simulink model "CryoDetXray"  (R2016b)
settings: Solver=ode45  StartTime=0.0  StopTime=10e-5  MaxStep=Tclk/4  RelTol=1e-3
values from neighbouring files (symbols this model uses):
  Fclk = Fadc    (= 307200000)    [setupCryoFPGAxray.m]
  Tclk = 1/Fclk    (= 3.25520833333e-09)    [setupCryoFPGAxray.m]
undefined symbols (not defined in the file or in its folder): AXI4, Lite, lpf, Naxi, xlipgetpartsetting
libraries: xbsIndex_r4 x1091, CryoDetLib x68, simulink x4, hdlsllib x1
(part 8 of 8)

== system CryoDetXray/DspCore/AdcDac 0/loopFilter1/initial Frequencies ==
  note: initial Frequencies
  note: select initial frequency
      | for now just mux from input registers
      | eventually configure RAM and loading protocol
  channel : Inport
  Gateway Out12 : xbsIndex_r4/Gateway Out  inherit_from_input=off  hdl_port=off  rows=1  columns=1  UseAsDAC=off  DACChannel='1'  interface=None  automatic_assignment=on  address_offset=hex2dec('00')  intf_name=''  intf_description=''  timing_constraint=None  locs_specified=off  LOCs={}  io_standard={}  block_type=gatewayout
  Gateway Out13 : xbsIndex_r4/Gateway Out  inherit_from_input=off  hdl_port=off  rows=1  columns=1  UseAsDAC=off  DACChannel='1'  interface=None  automatic_assignment=on  address_offset=hex2dec('00')  intf_name=''  intf_description=''  timing_constraint=None  locs_specified=off  LOCs={}  io_standard={}  block_type=gatewayout
  Mux : xbsIndex_r4/Mux  inputs=16  en=off  latency=0  precision=Full  arith_type=Unsigned  n_bits=24  bin_pt=24  quantization=Truncate  overflow=Wrap  dbl_ovrd=off  block_type=mux
  initial Freqs : Scope  NumInputPorts=2
  Fi : Outport
  wires:
  channel/1 -> Mux/1, Gateway Out12/1
  [F0] -> Mux/2
  [F1] -> Mux/3
  [F2] -> Mux/4
  [F3] -> Mux/5
  [F4] -> Mux/6
  [F5] -> Mux/7
  [F6] -> Mux/8
  [F7] -> Mux/9
  [F8] -> Mux/10
  [F9] -> Mux/11
  [F10] -> Mux/12
  [F11] -> Mux/13
  Mux/1 -> Gateway Out13/1, Fi/1
  Gateway Out13/1 -> initial Freqs/2
  Gateway Out12/1 -> initial Freqs/1
  [F12] -> Mux/14
  [F13] -> Mux/15
  [F14] -> Mux/16
  [F15] -> Mux/17

== system CryoDetXray/DspCore/AdcDac 0/16LineUDC 0/DAC Sum/DAC Q0 SUM ==
  note: Changed from 12 channel to 16 channels 8Sept2017
  In1 : Inport
  Bus Selector1 : BusSelector  OutputSignals=toDAC0.Q0,toDAC1.Q0,toDAC2.Q0,toDAC3.Q0,toDAC4.Q0,toDAC5.Q0,toDAC6.Q0,toDAC7.Q0,toDAC8.Q0,toDAC9.Q0,toDAC10.Q0,toDAC11.Q0,toDAC12.Q0,toDAC13.Q0,toDAC14.Q0,toDAC15.Q0
  DAC subSum : CryoDetLib/DAC subSum
  Out1 : Outport
  wires:
  In1/1 -> Bus Selector1/1
  Bus Selector1/1 -> DAC subSum/1  "<Q0>"
  Bus Selector1/16 -> DAC subSum/16  "<Q0>"
  DAC subSum/1 -> Out1/1
  Bus Selector1/2 -> DAC subSum/2  "<Q0>"
  Bus Selector1/3 -> DAC subSum/3  "<Q0>"
  Bus Selector1/4 -> DAC subSum/4  "<Q0>"
  Bus Selector1/5 -> DAC subSum/5  "<Q0>"
  Bus Selector1/6 -> DAC subSum/6  "<Q0>"
  Bus Selector1/7 -> DAC subSum/7  "<Q0>"
  Bus Selector1/8 -> DAC subSum/8  "<Q0>"
  Bus Selector1/9 -> DAC subSum/9  "<Q0>"
  Bus Selector1/10 -> DAC subSum/10  "<Q0>"
  Bus Selector1/11 -> DAC subSum/11  "<Q0>"
  Bus Selector1/12 -> DAC subSum/12  "<Q0>"
  Bus Selector1/13 -> DAC subSum/13  "<Q0>"
  Bus Selector1/14 -> DAC subSum/14  "<Q0>"
  Bus Selector1/15 -> DAC subSum/15  "<Q0>"

== system CryoDetXray/DspCore/AdcDac 0/16LineUDC 0/DAC Sum/DAC Q1 SUM ==
  note: Changed from 12 channel to 16 channels 8Sept2017
  note: Final adder stages
      | divide by 8
      | and reduce to 16 bits
  In1 : Inport
  Bus Selector1 : BusSelector  OutputSignals=toDAC0.Q1,toDAC1.Q1,toDAC2.Q1,toDAC3.Q1,toDAC4.Q1,toDAC5.Q1,toDAC6.Q1,toDAC7.Q1,toDAC8.Q1,toDAC9.Q1,toDAC10.Q1,toDAC11.Q1,toDAC12.Q1,toDAC13.Q1,toDAC14.Q1,toDAC15.Q1
  DAC subSum : CryoDetLib/DAC subSum
  Out1 : Outport
  wires:
  In1/1 -> Bus Selector1/1
  Bus Selector1/1 -> DAC subSum/1  "<Q1>"
  Bus Selector1/16 -> DAC subSum/16  "<Q1>"
  DAC subSum/1 -> Out1/1
  Bus Selector1/2 -> DAC subSum/2  "<Q1>"
  Bus Selector1/3 -> DAC subSum/3  "<Q1>"
  Bus Selector1/4 -> DAC subSum/4  "<Q1>"
  Bus Selector1/5 -> DAC subSum/5  "<Q1>"
  Bus Selector1/6 -> DAC subSum/6  "<Q1>"
  Bus Selector1/7 -> DAC subSum/7  "<Q1>"
  Bus Selector1/8 -> DAC subSum/8  "<Q1>"
  Bus Selector1/9 -> DAC subSum/9  "<Q1>"
  Bus Selector1/10 -> DAC subSum/10  "<Q1>"
  Bus Selector1/11 -> DAC subSum/11  "<Q1>"
  Bus Selector1/12 -> DAC subSum/12  "<Q1>"
  Bus Selector1/13 -> DAC subSum/13  "<Q1>"
  Bus Selector1/14 -> DAC subSum/14  "<Q1>"
  Bus Selector1/15 -> DAC subSum/15  "<Q1>"

== system CryoDetXray/DspCore/AdcDac 0/16LineUDC 0/DAC Sum/DAC i0 SUM ==
  note: Changed from 12 channel to 16 channels 8Sept2017
  In1 : Inport
  Bus Selector1 : BusSelector  OutputSignals=toDAC0.I0,toDAC1.I0,toDAC2.I0,toDAC3.I0,toDAC4.I0,toDAC5.I0,toDAC6.I0,toDAC7.I0,toDAC8.I0,toDAC9.I0,toDAC10.I0,toDAC11.I0,toDAC12.I0,toDAC13.I0,toDAC14.I0,toDAC15.I0
  DAC subSum : CryoDetLib/DAC subSum
  Out1 : Outport
  wires:
  In1/1 -> Bus Selector1/1
  Bus Selector1/1 -> DAC subSum/1  "<I0>"
  Bus Selector1/16 -> DAC subSum/16  "<I0>"
  DAC subSum/1 -> Out1/1
  Bus Selector1/2 -> DAC subSum/2  "<I0>"
  Bus Selector1/3 -> DAC subSum/3  "<I0>"
  Bus Selector1/4 -> DAC subSum/4  "<I0>"
  Bus Selector1/5 -> DAC subSum/5  "<I0>"
  Bus Selector1/6 -> DAC subSum/6  "<I0>"
  Bus Selector1/7 -> DAC subSum/7  "<I0>"
  Bus Selector1/8 -> DAC subSum/8  "<I0>"
  Bus Selector1/9 -> DAC subSum/9  "<I0>"
  Bus Selector1/10 -> DAC subSum/10  "<I0>"
  Bus Selector1/11 -> DAC subSum/11  "<I0>"
  Bus Selector1/12 -> DAC subSum/12  "<I0>"
  Bus Selector1/13 -> DAC subSum/13  "<I0>"
  Bus Selector1/14 -> DAC subSum/14  "<I0>"
  Bus Selector1/15 -> DAC subSum/15  "<I0>"

== system CryoDetXray/DspCore/AdcDac 0/16LineUDC 0/DAC Sum/DAC i1 SUM ==
  note: Changed from 12 channel to 16 channels 8Sept2017
  In1 : Inport
  Bus Selector1 : BusSelector  OutputSignals=toDAC0.I1,toDAC1.I1,toDAC2.I1,toDAC3.I1,toDAC4.I1,toDAC5.I1,toDAC6.I1,toDAC7.I1,toDAC8.I1,toDAC9.I1,toDAC10.I1,toDAC11.I1,toDAC12.I1,toDAC13.I1,toDAC14.I1,toDAC15.I1
  DAC subSum : CryoDetLib/DAC subSum
  Out1 : Outport
  wires:
  In1/1 -> Bus Selector1/1
  Bus Selector1/1 -> DAC subSum/1  "<I1>"
  Bus Selector1/16 -> DAC subSum/16  "<I1>"
  DAC subSum/1 -> Out1/1
  Bus Selector1/2 -> DAC subSum/2  "<I1>"
  Bus Selector1/3 -> DAC subSum/3  "<I1>"
  Bus Selector1/4 -> DAC subSum/4  "<I1>"
  Bus Selector1/5 -> DAC subSum/5  "<I1>"
  Bus Selector1/6 -> DAC subSum/6  "<I1>"
  Bus Selector1/7 -> DAC subSum/7  "<I1>"
  Bus Selector1/8 -> DAC subSum/8  "<I1>"
  Bus Selector1/9 -> DAC subSum/9  "<I1>"
  Bus Selector1/10 -> DAC subSum/10  "<I1>"
  Bus Selector1/11 -> DAC subSum/11  "<I1>"
  Bus Selector1/12 -> DAC subSum/12  "<I1>"
  Bus Selector1/13 -> DAC subSum/13  "<I1>"
  Bus Selector1/14 -> DAC subSum/14  "<I1>"
  Bus Selector1/15 -> DAC subSum/15  "<I1>"

== system CryoDetXray/DspCore/AdcDac 0/16LineUDC 0/SBdemod/CIC reset ==
  note: 29 Sep 2017
      | May need to rejigger logic for 307 MHz clock timing
  note: where N is number of channels in CIC filter
  note: reset latched resetIn
  note: latch resetIn
  note: CIC reset
      |
      | Synchronizes a CIC compiler 4.0 multi-channel CIC filter
      | to input channels
      |
      | Generates:
      | 1	notResetOut to CIC aresetn
      | 2	tlast to CIC tlast input
      |
      | Inputs:
      | 1	reset in
      | 2	Channel number (0-N) which may go to sel input of mux generating the input data stream
      | 3	N-2 which tells this module how deep is the multiplexing (e.g. N-2 = 10 for a 12 channel CIC filter (sorry))
      |
      | Guarantees:
      | 1	reset out is at least 2 clocks long
      | 2	end of reset occurs 2 clocks before channel 0
      | 3	tlast comes with channel N-1
      |
      | Assumes:
      | CIC oversampling set to "Sample period" = 1
      | No "streaming interface"
  resetIn : Inport
  Channel : Inport  Port=2
  N-2 : Inport  Port=3
  Constant : xbsIndex_r4/Constant  const=0  gui_display_data_type=Boolean  arith_type=Boolean  n_bits=16  bin_pt=14  preci_type=Single  exp_width=8  frac_width=24  explicit_period=off  period=1  equ=P=C  opselect=C  inp2=PCIN>>17  opr=+  inp1=P  carry=CIN  dbl_ovrd=off  block_type=constant
  Delay1 : xbsIndex_r4/Delay  rst=off  infoeditControl=Selection of Reset will increase slice count due to use of real FFs and instead of SRLs  en=off  latency=1  reg_retiming=off  dbl_ovrd=off  block_type=delay
  Delay2 : xbsIndex_r4/Delay  rst=off  infoeditControl=Selection of Reset will increase slice count due to use of real FFs and instead of SRLs  en=off  latency=1  reg_retiming=on  dbl_ovrd=off  block_type=delay
  Delay3 : xbsIndex_r4/Delay  rst=off  infoeditControl=Selection of Reset will increase slice count due to use of real FFs and instead of SRLs  en=off  latency=1  reg_retiming=on  dbl_ovrd=off  block_type=delay
  Inverter : xbsIndex_r4/Inverter  en=off  latency=2  dbl_ovrd=off  block_type=inv
  Inverter1 : xbsIndex_r4/Inverter  en=off  latency=0  dbl_ovrd=off  block_type=inv
  Logical : xbsIndex_r4/Logical  logical_function=AND  inputs=4  en=off  latency=0  precision=User Defined  arith_type=Boolean  n_bits=1  bin_pt=0  align_bp=on  dbl_ovrd=off  block_type=logical
  Logical1 : xbsIndex_r4/Logical  logical_function=OR  inputs=2  en=off  latency=0  precision=User Defined  arith_type=Boolean  n_bits=1  bin_pt=0  align_bp=on  dbl_ovrd=off  block_type=logical
  Mux : xbsIndex_r4/Mux  inputs=2  en=off  latency=0  precision=Full  arith_type=Unsigned  n_bits=16  bin_pt=14  quantization=Truncate  overflow=Wrap  dbl_ovrd=off  block_type=mux
  Relational1 : xbsIndex_r4/Relational  mode=a=b  op_type=Bool  en=off  latency=0  dbl_ovrd=off  block_type=relational
  notResetOut : Outport
  tlast : Outport  Port=2
  wires:
  resetIn/1 -> Inverter/1, Logical1/1
  Channel/1 -> Relational1/1
  N-2/1 -> Relational1/2
  Relational1/1 -> Logical/4, Delay1/1
  Logical1/1 -> Inverter1/1, Delay2/1
  Mux/1 -> Logical1/2
  Delay2/1 -> Logical/2, Delay3/1, Mux/2
  Constant/1 -> Mux/3
  Logical/1 -> Mux/1
  Delay1/1 -> tlast/1
  Inverter/1 -> Logical/1
  Delay3/1 -> Logical/3
  Inverter1/1 -> notResetOut/1

== system CryoDetXray/DspCore/AdcDac 0/S21/Complex Divide/CplxProd ==
  tvalidIn : Inport
  Im_A : Inport  Port=2
  Re_A : Inport  Port=3
  Im_B : Inport  Port=4
  Re_B : Inport  Port=5
  AddSub : xbsIndex_r4/AddSub  mode=Subtraction  use_carryin=off  use_carryout=off  en=off  latency=4  precision=Full  arith_type=Unsigned  n_bits=16  bin_pt=14  quantization=Truncate  overflow=Wrap  use_behavioral_HDL=off  hw_selection=Fabric  pipelined=off  dbl_ovrd=off  block_type=addsub
  AddSub1 : xbsIndex_r4/AddSub  mode=Addition  use_carryin=off  use_carryout=off  en=off  latency=4  precision=Full  arith_type=Unsigned  n_bits=16  bin_pt=14  quantization=Truncate  overflow=Wrap  use_behavioral_HDL=off  hw_selection=Fabric  pipelined=off  dbl_ovrd=off  block_type=addsub
  Delay : xbsIndex_r4/Delay  rst=off  infoeditControl=Selection of Reset will increase slice count due to use of real FFs and instead of SRLs  en=off  latency=4  reg_retiming=on  dbl_ovrd=off  block_type=delay
  Delay1 : xbsIndex_r4/Delay  rst=off  infoeditControl=Selection of Reset will increase slice count due to use of real FFs and instead of SRLs  en=off  latency=3  reg_retiming=on  dbl_ovrd=off  block_type=delay
  Mult : xbsIndex_r4/Mult  precision=Full  arith_type="Signed  (2's comp)"  n_bits=16  bin_pt=14  quantization=Truncate  overflow=Wrap  en=off  latency=4  use_behavioral_HDL=off  opt=Speed  use_embedded=on  optimum_pipeline=on  pipeline=on  dbl_ovrd=off  use_rpm=on  placement_style=Triangular  block_type=mult
  Mult1 : xbsIndex_r4/Mult  precision=Full  arith_type="Signed  (2's comp)"  n_bits=16  bin_pt=14  quantization=Truncate  overflow=Wrap  en=off  latency=4  use_behavioral_HDL=off  opt=Speed  use_embedded=on  optimum_pipeline=on  pipeline=on  dbl_ovrd=off  use_rpm=on  placement_style=Triangular  block_type=mult
  Mult2 : xbsIndex_r4/Mult  precision=Full  arith_type="Signed  (2's comp)"  n_bits=16  bin_pt=14  quantization=Truncate  overflow=Wrap  en=off  latency=4  use_behavioral_HDL=off  opt=Speed  use_embedded=on  optimum_pipeline=off  pipeline=on  dbl_ovrd=off  use_rpm=on  placement_style=Triangular  block_type=mult
  Mult3 : xbsIndex_r4/Mult  precision=Full  arith_type="Signed  (2's comp)"  n_bits=16  bin_pt=14  quantization=Truncate  overflow=Wrap  en=off  latency=4  use_behavioral_HDL=off  opt=Speed  use_embedded=on  optimum_pipeline=off  pipeline=on  dbl_ovrd=off  use_rpm=on  placement_style=Triangular  block_type=mult
  tvalidOut : Outport
  Im_Out : Outport  Port=2
  Re_Out : Outport  Port=3
  wires:
  Delay/1 -> Delay1/1
  Mult2/1 -> AddSub1/1
  Mult/1 -> AddSub/1
  Mult1/1 -> AddSub/2
  Mult3/1 -> AddSub1/2
  Re_A/1 -> Mult3/1, Mult/1
  Im_A/1 -> Mult2/1, Mult1/1
  tvalidIn/1 -> Delay/1
  Im_B/1 -> Mult1/2, Mult3/2
  Re_B/1 -> Mult/2, Mult2/2
  Delay1/1 -> tvalidOut/1
  AddSub/1 -> Re_Out/1
  AddSub1/1 -> Im_Out/1
